simulink model "Circuit_Model"  (R2016a)
settings: Solver=VariableStepAuto  StartTime=0.0  StopTime=0.25  RelTol=1e-3
libraries: pe_lib x17, fl_lib x10, nesl_utility x3, elec_lib x1
settings Model: Creator=Rohith  LastModifiedBy=Rohith

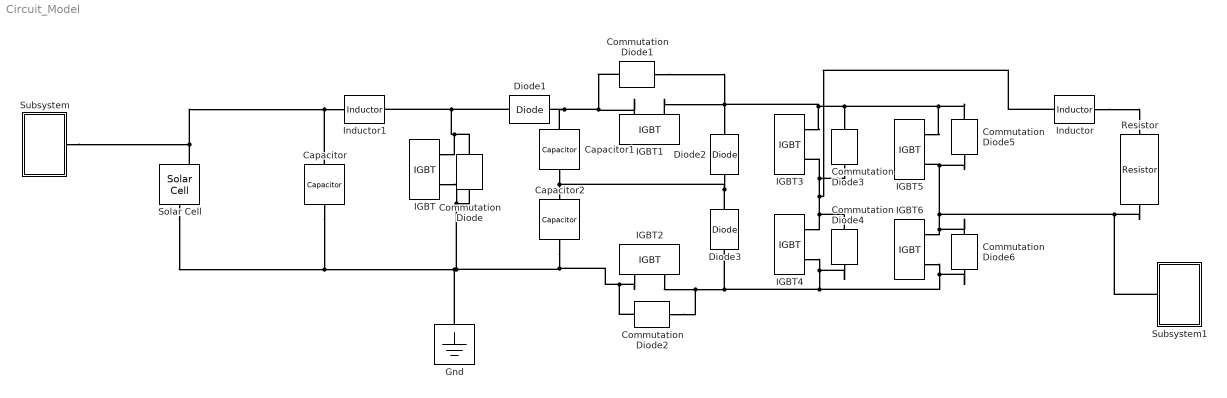
== system Circuit_Model ==
  Capacitor : fl_lib/Electrical/Electrical Elements/Capacitor  c=470 uF  r=1e-6 Ohm  g=0 1/Ohm  i_specify=off  i_priority=None  i=0 A  v_specify=off  v_priority=None  v=0 V  vc_specify=off  vc_priority=High  vc=0 V
  Capacitor1 : fl_lib/Electrical/Electrical Elements/Capacitor  c=2200 uF  r=1e-6 Ohm  g=0 1/Ohm  i_specify=off  i_priority=None  i=0 A  v_specify=off  v_priority=None  v=0 V  vc_specify=off  vc_priority=High  vc=0 V
  Capacitor2 : fl_lib/Electrical/Electrical Elements/Capacitor  c=2200 uF  r=1e-6 Ohm  g=0 1/Ohm  i_specify=off  i_priority=None  i=0 A  v_specify=off  v_priority=None  v=0 V  vc_specify=off  vc_priority=High  vc=0 V
  Commutation Diode{,1..6} (7 alike) : pe_lib/Semiconductors/Fundamental Components/Commutation Diode  Vf=0.8 V  Ron=0.001 Ohm  Goff=1e-5 1/Ohm  N_series=1  N_parallel=1  C=50 nF  iRM=-235 A  iF=300 A  idot=-50 A/us  trr_param=1  trr_factor=3  trr=15 us  Qrr=1.5e+3 s*uA
  Diode1 : pe_lib/Semiconductors/Fundamental Components/Diode  Vf=0.8 V  Ron=0.001 Ohm  Goff=1e-5 1/Ohm  N_series=1  N_parallel=1  Vf_equiv=0.8 V  Ron_equiv=0.001 Ohm  Goff_equiv=1e-5 1/Ohm
  Diode2 : pe_lib/Semiconductors/Fundamental Components/Diode  Vf=0.8 V  Ron=0.001 Ohm  Goff=1e-5 1/Ohm  N_series=1  N_parallel=1  Vf_equiv=0.8 V  Ron_equiv=0.001 Ohm  Goff_equiv=1e-5 1/Ohm
  Diode3 : pe_lib/Semiconductors/Fundamental Components/Diode  Vf=0.8 V  Ron=0.001 Ohm  Goff=1e-5 1/Ohm  N_series=1  N_parallel=1  Vf_equiv=0.8 V  Ron_equiv=0.001 Ohm  Goff_equiv=1e-5 1/Ohm
  Gnd : fl_lib/Electrical/Electrical Elements/Electrical Reference
  IGBT{,1..6} (7 alike) : pe_lib/Semiconductors/Fundamental Components/IGBT  Vf=0.8 V  Ron=0.001 Ohm  Goff=1e-5 1/Ohm  Vth=6 V  diode_param=1  diode_Vf=0.8 V  diode_Ron=0.001 Ohm  diode_Goff=1e-5 1/Ohm  diode_C=5e-8 F  diode_iRM=-235 A  diode_iF=300 A  diode_idot=-50 A/us  diode_trr_param=1  diode_trr_factor=3  diode_trr=15 us  diode_Qrr=1.5e+3 s*uA  thermal_loss_option=2  Voff=300 V  Tau=1e-4 s  Tj=[ 298.15 398.15 ] K  Iout_data=[ 0 10 50 100 200 400 600 ] A  Eon_data=[ 0 2.9e-4 0.00143 0.00286 0.00571 0.01314 0.02286; 0 5.7e-4 0.00263 0.00514 0.01029 0.02057 0.03029 ] J  Eoff_data=[ 0 2.1e-4 0.00107 0.00214 0.00429 0.009859999999999999 0.01714; 0 4.3e-4 0.00197 0.00386 0.00771 0.01543 0.02271 ] J  Von_data=[ 0 1.1 1.3 1.45 1.75 2.25 2.7; 0 1 1.15 1.35 1.7 2.35 3 ] V
  Inductor : fl_lib/Electrical/Electrical Elements/Inductor  l=1.4 mH  r=0 Ohm  g=1e-9 1/Ohm  i_specify=off  i_priority=None  i=0 A  v_specify=off  v_priority=None  v=0 V  i_L_specify=off  i_L_priority=High  i_L=0 A
  Inductor1 : fl_lib/Electrical/Electrical Elements/Inductor  l=2 mH  r=0 Ohm  g=1e-9 1/Ohm  i_specify=off  i_priority=None  i=0 A  v_specify=off  v_priority=None  v=0 V  i_L_specify=off  i_L_priority=High  i_L=0 A
  Resistor : fl_lib/Electrical/Electrical Elements/Resistor  R=1 MOhm  i_specify=off  i_priority=None  i=0 A  v_specify=off  v_priority=None  v=0 V
  Solar Cell : elec_lib/Sources/Solar Cell  prm=1  Isc=5 A  Voc=21.7 V  Is=1e-6 A  Is2=0 A  Iph=7.34 A  Ir0=1000 W/m^2  ec=1.5  N2=2  Rs=0 Ohm  Rp=Inf Ohm  N_series=1  TIPH1=0 1/K  EG=1.11 eV  TXIS1=3  TXIS2=3  TRS1=0  TRP1=0  Tmeas=25 degC  TFIXED=25 degC  thermal_mass=100 J/K  initial_temperature=25 degC
  Subsystem : Subsystem
  Subsystem1 : Subsystem
  connections:
  Diode1/LConn1 -- Commutation Diode/RConn1 -- IGBT/RConn1 -- Inductor1/RConn1
  IGBT1/RConn1 -- Commutation Diode1/RConn1 -- Capacitor1/LConn1 -- Diode1/RConn1
  Capacitor1/RConn1 -- Diode3/RConn1 -- Diode2/LConn1 -- Capacitor2/LConn1
  IGBT/RConn2 -- Gnd/LConn1 -- Capacitor/RConn1 -- Solar Cell/RConn1 -- IGBT2/RConn2 -- Commutation Diode2/LConn1 -- Capacitor2/RConn1 -- Commutation Diode/LConn1
  IGBT1/RConn2 -- Commutation Diode5/RConn1 -- IGBT5/RConn1 -- Commutation Diode3/RConn1 -- IGBT3/RConn1 -- Commutation Diode1/LConn1 -- Diode2/RConn1
  IGBT2/RConn1 -- Commutation Diode2/RConn1 -- Commutation Diode6/LConn1 -- IGBT6/RConn2 -- Commutation Diode4/LConn1 -- IGBT4/RConn2 -- Diode3/LConn1
  IGBT4/RConn1 -- Commutation Diode4/RConn1 -- Inductor/LConn1 -- Commutation Diode3/LConn1 -- IGBT3/RConn2
  IGBT6/RConn1 -- Commutation Diode6/RConn1 -- Subsystem1/LConn1 -- Resistor/RConn1 -- Commutation Diode5/LConn1 -- IGBT5/RConn2
  Capacitor/LConn1 -- Subsystem/LConn1 -- Solar Cell/LConn2 -- Inductor1/LConn1
  Inductor/RConn1 -- Resistor/LConn1

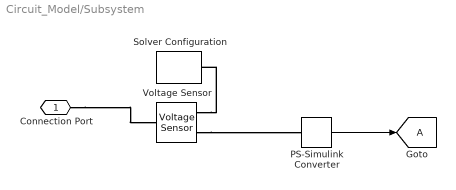
== system Circuit_Model/Subsystem ==
  PS-Simulink Converter : nesl_utility/PS-Simulink Converter  PhysicalDomain=network_engine_domain  SubClassName=ps_output  LeftPortType=input  RightPortType=output  PseudoPeriodic=off  Frequencies=[]  Unit=1  AffineConversion=off
  Solver Configuration : nesl_utility/Solver Configuration  PhysicalDomain=network_engine_domain  SubClassName=solver  LeftPortType=input  RightPortType=generic  Accelerate=off  Tones=[]  Harmonics=[]  SimulateNoise=off  Profile=off  UseLocalSampling=off  EnableSwitchedLinearOptims=on  FrequencyDomain=off  UseCCode=off  RelTol=0.001  AbsTol=1e-06  MinStep=1e-09  ToWorkspace=off  RevertToSquareIcSolve=off  NumHomotopyIterations=100  PhasorMode=off  PhasorModeNumHarmonics=1  OverrideAbsTol=off  DoDC=off  ResidualTolerance=1e-09  UseLocalSolver=off  LocalSolverChoice=NE_BACKWARD_EULER_ADVANCER  LocalSolverSampleTime=0.001  DoFixedCost=off  MaxNonlinIter=3  MaxModeIter=2  LinearAlgebra=Sparse  DelaysMemoryBudget=1024  AutomaticFiltering=on  FilteringTimeConstant=0.001
  Voltage Sensor : fl_lib/Electrical/Electrical Sensors/Voltage Sensor
  Connection Port : PMIOPort  Port=1  Side=Left
  tag scope: A=global
  wires:
  PS-Simulink Converter/1 -> [A]
  connections:
  Voltage Sensor/RConn1 -- PS-Simulink Converter/LConn1
  Connection Port/RConn1 -- Voltage Sensor/LConn1
  Voltage Sensor/RConn2 -- Solver Configuration/RConn1

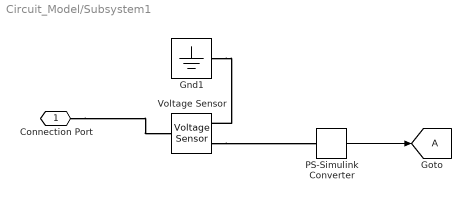
== system Circuit_Model/Subsystem1 ==
  Gnd1 : fl_lib/Electrical/Electrical Elements/Electrical Reference
  PS-Simulink Converter : nesl_utility/PS-Simulink Converter  PhysicalDomain=network_engine_domain  SubClassName=ps_output  LeftPortType=input  RightPortType=output  PseudoPeriodic=off  Frequencies=[]  Unit=1  AffineConversion=off
  Voltage Sensor : fl_lib/Electrical/Electrical Sensors/Voltage Sensor
  Connection Port : PMIOPort  Port=1  Side=Left
  tag scope: A=global
  wires:
  PS-Simulink Converter/1 -> [A]
  connections:
  Gnd1/LConn1 -- Voltage Sensor/RConn2
  Connection Port/RConn1 -- Voltage Sensor/LConn1
  Voltage Sensor/RConn1 -- PS-Simulink Converter/LConn1
